simulink model "model_zad3"  (Simulink 8.0)
settings: Solver=ode4  StartTime=0.0  StopTime=30.0  FixedStep=0.01  RelTol=1e-3
values from neighbouring files (symbols this model uses):
  Amplituda = Amps(i)    [Jakub_Adamczyk_skrypt.m]
  Czestotliwosc = Freqs(i)    [Jakub_Adamczyk_skrypt.m]
  Faza = fis(i)    [Jakub_Adamczyk_skrypt.m]
  Licznik = [1]    [Jakub_Adamczyk_skrypt.m]
  Mianownik = [T, 1]    [Jakub_Adamczyk_skrypt.m]
settings Model: Creator=Jakub Adamczyk  LastModifiedBy=Jakub Adamczyk

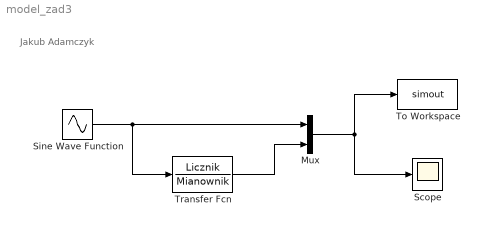
== system model_zad3 ==
  note: Jakub Adamczyk
  Mux : Mux  Inputs=2
  Scope : Scope
  Sine Wave Function : Sin  Amplitude=Amplituda  Frequency=Czestotliwosc  Phase=Faza  SampleTime=0
  To Workspace : ToWorkspace  VariableName=simout  SampleTime=-1
  Transfer Fcn : TransferFcn  Numerator=Licznik  Denominator=Mianownik
  wires:
  Sine Wave Function/1 -> Transfer Fcn/1, Mux/1
  Transfer Fcn/1 -> Mux/2
  Mux/1 -> To Workspace/1, Scope/1
